simulink model "neckVel"  (Simulink 8.0)
settings: Solver=FixedStepDiscrete  StartTime=0.0  StopTime=inf  FixedStep=Ts  RelTol=1e-3
InitFcn:
  | initNeckVel;
undefined symbols (not defined in the file): DiscIntNeverNeededParam, DT, kCom, kImp, kw, qFin, Ts
libraries: WBCLibrary x36
settings Model: Creator=daniele  LastModifiedBy=icub
settings DebuggingCC: FcnCallInpInsideContextMsg=EnableAllAsWarning
settings CodeAppCC: CustomSymbolStrType=$N$R$M_T
settings GRTTargetCC: CodeReplacementLibrary=C89/C90 (ANSI)  CombineOutputUpdateFcns=off  GRTInterface=on

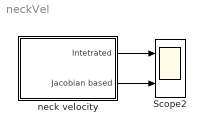
== system neckVel ==
  Scope2 : Scope  NumInputPorts=2
      settings: ShowLegends=on  YMin=-15~-5  YMax=70~5  SaveName=ScopeData2
  neck velocity : Subsystem  mask{robotName='icubGazeboSim', localName='simulink', Ts=Ts}
      mask prompts: robotName "Robot name"; localName "Local name"
  wires:
  neck velocity/1(Intetrated) -> Scope2/1
  neck velocity/2(Jacobian based) -> Scope2/2

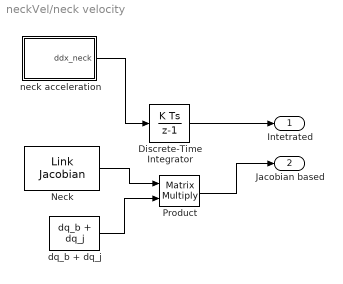
== system neckVel/neck velocity ==
  Discrete-Time Integrator : DiscreteIntegrator  InitialCondition=[0 0 0 0 0 0]  SampleTime=Ts  ICPrevOutput=DiscIntNeverNeededParam  ICPrevScaledInput=DiscIntNeverNeededParam
  Neck : WBCLibrary/wholeBodyModel/Jacobians/Link Jacobian  robotname=robotName  localname=localName  link=chest
  Product : Product  Multiplication=Matrix(*)  SampleTime=Ts  RndMeth=Zero
  dq_b + dq_j : WBCLibrary/wholeBodyStates/dq_b + dq_j  robotName=robotName  localName=localName  Ts=Ts
  neck acceleration : Subsystem  mask{robotName=robotName, localName=localName, Ts=0.010}
      mask prompts: robotName "Robot name"; localName "Local name"
  Intetrated : Outport
  Jacobian based : Outport  Port=2
  wires:
  dq_b + dq_j/1 -> Product/2
  Neck/1 -> Product/1
  Product/1 -> Jacobian based/1
  neck acceleration/1(ddx_neck) -> Discrete-Time Integrator/1
  Discrete-Time Integrator/1 -> Intetrated/1

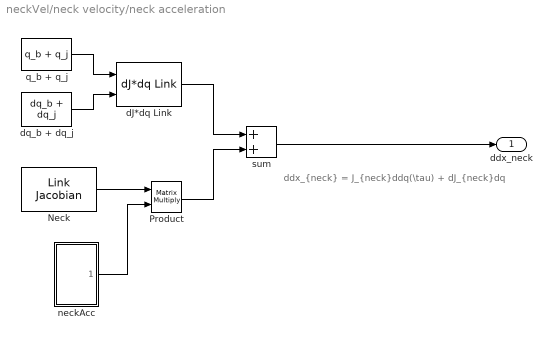
== system neckVel/neck velocity/neck acceleration ==
  note: ddx_{neck} = J_{neck}ddq(\tau) + dJ_{neck}dq
  Neck : WBCLibrary/wholeBodyModel/Jacobians/Link Jacobian  robotname=robotName  localname=localName  link=chest
  Product : Product  Multiplication=Matrix(*)  RndMeth=Zero
  dJ*dq Link : WBCLibrary/wholeBodyModel/Dynamics/dJ*dq Link  val=19  robotName=robotName  localName=localName  link=chest
  dq_b + dq_j : WBCLibrary/wholeBodyStates/dq_b + dq_j  robotName=robotName  localName=localName  Ts=Ts
  neckAcc : Subsystem  mask{robotName=robotName, Ts=Ts, localName=localName}
      mask prompts: robotName "robot name"; localName "module name"
  q_b + q_j : WBCLibrary/wholeBodyStates/q_b + q_j  robotName=robotName  localName=localName  Ts=Ts
  sum : Sum  SampleTime=Ts
  ddx_neck : Outport
  wires:
  dJ*dq Link/1 -> sum/1
  sum/1 -> ddx_neck/1
  q_b + q_j/1 -> dJ*dq Link/1
  neckAcc/1(ddq(tau)) -> Product/2
  Product/1 -> sum/2
  Neck/1 -> Product/1
  dq_b + dq_j/1 -> dJ*dq Link/2

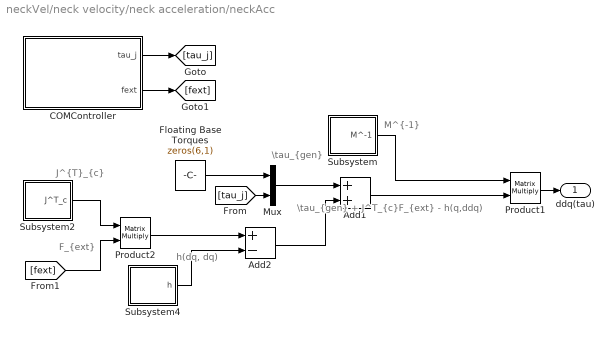
== system neckVel/neck velocity/neck acceleration/neckAcc ==
  note: \tau_{gen} + J^T_{c}F_{ext} - h(q,ddq)
  note: h(dq, dq)
  note: J^{T}_{c}
  note: M^{-1}
  note: F_{ext}
  note: \tau_{gen}
  Add1 : Sum  SampleTime=Ts
  Add2 : Sum  Inputs=+-  SampleTime=Ts
  COMController : Subsystem
  Floating Base Torques : Constant  Value=zeros(6,1)  SampleTime=Ts
  Mux : Mux  Inputs=2
  Product1 : Product  Multiplication=Matrix(*)  SampleTime=Ts
  Product2 : Product  Multiplication=Matrix(*)  SampleTime=Ts
  Subsystem : Subsystem
  Subsystem2 : Subsystem
  Subsystem4 : Subsystem
  ddq(tau) : Outport
  wires:
  Subsystem2/1(J^T_c) -> Product2/1
  [fext] -> Product2/2
  Product2/1 -> Add2/1
  Product1/1 -> ddq(tau)/1
  Add2/1 -> Add1/2
  Subsystem/1(M^-1) -> Product1/1
  Subsystem4/1(h) -> Add2/2
  Add1/1 -> Product1/2
  COMController/1(tau_j) -> [tau_j]
  COMController/2(fext) -> [fext]
  Floating Base Torques/1 -> Mux/1
  [tau_j] -> Mux/2
  Mux/1 -> Add1/1

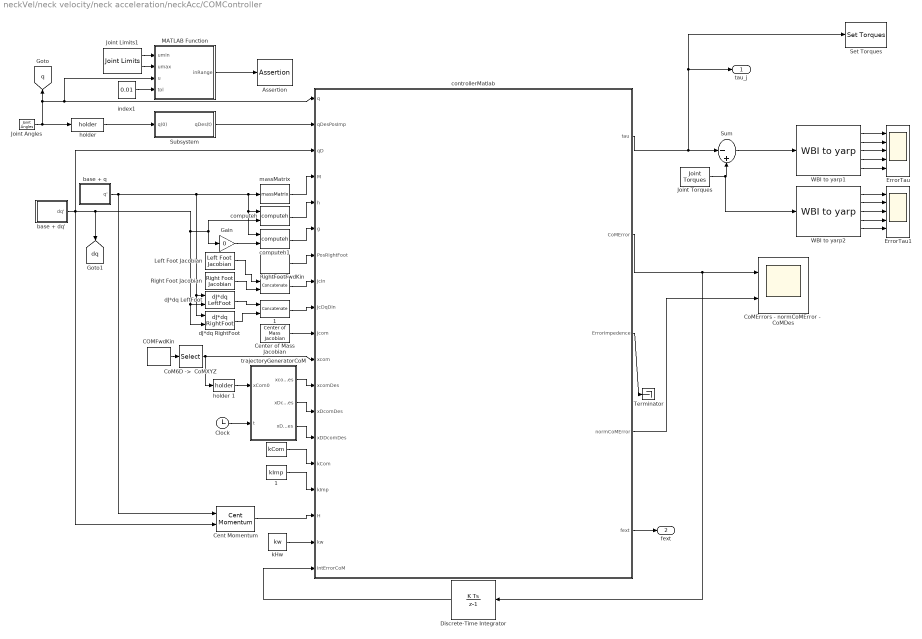
== system neckVel/neck velocity/neck acceleration/neckAcc/COMController ==
  "    " : Constant  Value=kCom
  "    1" : Constant  Value=kImp
  " " : Concatenate  Mode=Multidimensional array
  " 1" : Concatenate  Mode=Multidimensional array
  Assertion : Assertion  Enabled=on
  "COMFwdKin " : WBCLibrary/wholeBodyModel/Forward Kinematics/COMFwdKin   robotName=robotName  localName=localName
  Cent Momentum : WBCLibrary/wholeBodyModel/Dynamics/Cent Momentum  robotName=robotName  localName=localName
  Center of Mass Jacobian : WBCLibrary/wholeBodyModel/Jacobians/Center of Mass Jacobian  robotName=robotName  localName=localName
  Clock : Clock
  "CoM6D ->  CoMXYZ" : Selector  InputPortWidth=7  IndexOptions=Index vector (dialog)  Indices=[1 2 3]  OutputSizes=1
  "CoMErrors - normCoMError -   CoMDes " : Scope  NumInputPorts=2
      settings: TimeRange=0.5  YMin=-0.025~0  YMax=0.005~0.04  SaveName=ScopeData6
  Discrete-Time Integrator : DiscreteIntegrator  InitialCondition=[0 0 0]  SampleTime=Ts  ICPrevOutput=DiscIntNeverNeededParam  ICPrevScaledInput=DiscIntNeverNeededParam
  ErrorTau : Scope  NumInputPorts=5
      settings: ShowLegends=on  YMin=-12~-5~-5~-5~-5  YMax=12~5~5~5~5
  ErrorTau1 : Scope  NumInputPorts=5
      settings: YMin=-12~-5~-5~-5~-5  YMax=12~5~5~5~5
  Gain : Gain  Gain=0
  Joint Angles : WBCLibrary/wholeBodyStates/Joint Angles  robotName=robotName  localName=localName
  Joint Limits1 : WBCLibrary/wholeBodyModel/Joint Limits  robotName=robotName  localName=localName
  Joint Torques : WBCLibrary/wholeBodyStates/Joint Torques  robotName=robotName  localName=localName
  Left Foot Jacobian : WBCLibrary/wholeBodyModel/Jacobians/Left Foot Jacobian  robotName=robotName  localName=localName
  MATLAB Function : MATLAB Function  TreatAsAtomicUnit=on
  Right Foot Jacobian : WBCLibrary/wholeBodyModel/Jacobians/Right Foot Jacobian  robotName=robotName  localName=localName
  RightFootFwdKin : WBCLibrary/wholeBodyModel/Forward Kinematics/RightFootFwdKin  robotName=robotName  localName=localName
  Set Torques : WBCLibrary/wholeBodyActuators/Set Torques  val=6  robotName=robotName  localName=localName
  Subsystem : Subsystem
  Sum : Sum  Inputs=|-+
  Terminator : Terminator
  WBI to yarp1 : WBCLibrary/Utilities/WBI to yarp
  WBI to yarp2 : WBCLibrary/Utilities/WBI to yarp
  base + dq' : Subsystem
  base + q : Subsystem
  computeh : WBCLibrary/wholeBodyModel/Dynamics/computeh  val=7  robotname=robotName  localname=localName
  computeh1 : WBCLibrary/wholeBodyModel/Dynamics/computeh  val=7  robotname=robotName  localname=localName
  controllerMatlab : MATLAB Function  TreatAsAtomicUnit=on
  dJ*dq LeftFoot : WBCLibrary/wholeBodyModel/Dynamics/dJ*dq LeftFoot  val=9  robotName=robotName  localName=localName
  dJ*dq RightFoot : WBCLibrary/wholeBodyModel/Dynamics/dJ*dq RightFoot  val=9  robotName=robotName  localName=localName
  "holder " : WBCLibrary/Utilities/holder 
  holder 1 : WBCLibrary/Utilities/holder 
  index1 : Constant  Value=0.01  VectorParams1D=off
  kHw : Constant  Value=kw
  massMatrix : WBCLibrary/wholeBodyModel/Dynamics/massMatrix  val=8  robotname=robotName  localname=localName
  trajectoryGeneratorCoM : MATLAB Function  TreatAsAtomicUnit=on
  tau_j : Outport
  fext : Outport  Port=2
  tag scope: dq=global, q=global
  wires:
  computeh/1 -> controllerMatlab/5(h)
  " "/1 -> controllerMatlab/8(JcIn)
  dJ*dq RightFoot/1 -> " 1"/2
  "    1"/1 -> controllerMatlab/16(kImp)
  kHw/1 -> controllerMatlab/18(kw)
  Joint Torques/1 -> WBI to yarp2/1, Sum/2
  WBI to yarp2/2 -> ErrorTau1/2
  MATLAB Function/1(inRange) -> Assertion/1
  "    "/1 -> controllerMatlab/15(kCom)
  WBI to yarp1/5 -> ErrorTau/5
  "CoM6D ->  CoMXYZ"/1 -> holder 1/1, controllerMatlab/11(xcom)
  base + q/1(q') -> dJ*dq RightFoot/1, dJ*dq LeftFoot/1, computeh1/1, computeh/1, massMatrix/1, Cent Momentum/1
  dJ*dq LeftFoot/1 -> " 1"/1
  base + dq'/1(dq') -> [dq], dJ*dq RightFoot/2, dJ*dq LeftFoot/2, computeh/2, Gain/1, Cent Momentum/2, controllerMatlab/3(qD)
  index1/1 -> MATLAB Function/4(tol)
  Joint Limits1/1 -> MATLAB Function/1(umin)
  "holder "/1 -> Subsystem/1(q(0))
  Gain/1 -> computeh1/2
  trajectoryGeneratorCoM/3(xDDcomDes) -> controllerMatlab/14(xDDcomDes)
  Subsystem/1(qDes(t)) -> controllerMatlab/2(qDesPosImp)
  WBI to yarp2/1 -> ErrorTau1/1
  computeh1/1 -> controllerMatlab/6(g)
  Joint Limits1/2 -> MATLAB Function/2(umax)
  WBI to yarp1/2 -> ErrorTau/2
  holder 1/1 -> trajectoryGeneratorCoM/1(xCom0)
  Clock/1 -> trajectoryGeneratorCoM/2(t)
  "COMFwdKin "/1 -> "CoM6D ->  CoMXYZ"/1
  Sum/1 -> WBI to yarp1/1
  trajectoryGeneratorCoM/1(xcomDes) -> controllerMatlab/12(xcomDes)
  Left Foot Jacobian/1 -> " "/1
  WBI to yarp2/4 -> ErrorTau1/4
  WBI to yarp1/3 -> ErrorTau/3
  massMatrix/1 -> controllerMatlab/4(M)
  WBI to yarp1/4 -> ErrorTau/4
  RightFootFwdKin/1 -> controllerMatlab/7(PosRightFoot)
  controllerMatlab/1(tau) -> tau_j/1, Set Torques/1, Sum/1
  trajectoryGeneratorCoM/2(xDcomDes) -> controllerMatlab/13(xDcomDes)
  Discrete-Time Integrator/1 -> controllerMatlab/19(IntErrorCoM)
  WBI to yarp1/1 -> ErrorTau/1
  Joint Angles/1 -> MATLAB Function/3(u), controllerMatlab/1(q), [q], "holder "/1
  WBI to yarp2/3 -> ErrorTau1/3
  controllerMatlab/4(normCoMError) -> "CoMErrors - normCoMError -   CoMDes "/2
  " 1"/1 -> controllerMatlab/9(JcDqDIn)
  Cent Momentum/1 -> controllerMatlab/17(H)
  controllerMatlab/2(CoMError) -> Discrete-Time Integrator/1, "CoMErrors - normCoMError -   CoMDes "/1
  controllerMatlab/3(ErrorImpedence) -> Terminator/1
  Center of Mass Jacobian/1 -> controllerMatlab/10(Jcom)
  Right Foot Jacobian/1 -> " "/2
  WBI to yarp2/5 -> ErrorTau1/5
  controllerMatlab/5(fext) -> fext/1

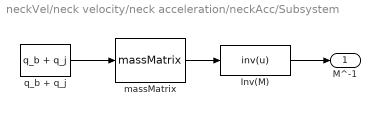
== system neckVel/neck velocity/neck acceleration/neckAcc/Subsystem ==
  Inv(M) : MATLABFcn  MATLABFcn=inv(u)  Output1D=off  SampleTime=Ts
  massMatrix : WBCLibrary/wholeBodyModel/Dynamics/massMatrix  val=8  robotname=robotName  localname=localName
  q_b + q_j : WBCLibrary/wholeBodyStates/q_b + q_j  robotName=robotName  localName=localName  Ts=Ts
  M^-1 : Outport
  wires:
  q_b + q_j/1 -> massMatrix/1
  Inv(M)/1 -> M^-1/1
  massMatrix/1 -> Inv(M)/1

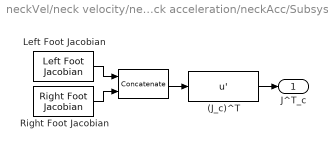
== system neckVel/neck velocity/neck acceleration/neckAcc/Subsystem2 ==
  " " : Concatenate  Mode=Multidimensional array
  (J_c)^T : MATLABFcn  MATLABFcn=u'  Output1D=off  SampleTime=Ts
  Left Foot Jacobian : WBCLibrary/wholeBodyModel/Jacobians/Left Foot Jacobian  robotName=robotName  localName=localName
  Right Foot Jacobian : WBCLibrary/wholeBodyModel/Jacobians/Right Foot Jacobian  robotName=robotName  localName=localName
  J^T_c : Outport
  wires:
  (J_c)^T/1 -> J^T_c/1
  " "/1 -> (J_c)^T/1
  Right Foot Jacobian/1 -> " "/2
  Left Foot Jacobian/1 -> " "/1

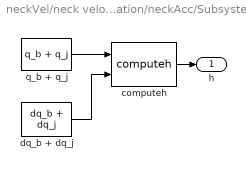
== system neckVel/neck velocity/neck acceleration/neckAcc/Subsystem4 ==
  computeh : WBCLibrary/wholeBodyModel/Dynamics/computeh  val=7  robotname=robotName  localname=localName
  dq_b + dq_j : WBCLibrary/wholeBodyStates/dq_b + dq_j  robotName=robotName  localName=localName  Ts=Ts
  q_b + q_j : WBCLibrary/wholeBodyStates/q_b + q_j  robotName=robotName  localName=localName  Ts=Ts
  h : Outport
  wires:
  computeh/1 -> h/1
  q_b + q_j/1 -> computeh/1
  dq_b + dq_j/1 -> computeh/2

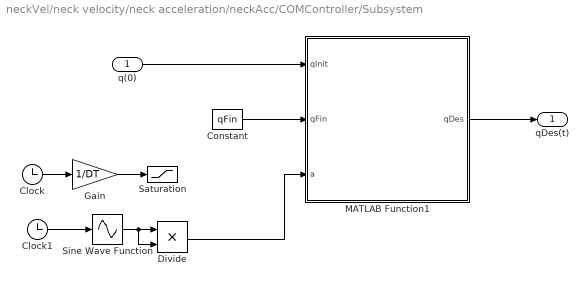
== system neckVel/neck velocity/neck acceleration/neckAcc/COMController/Subsystem ==
  q(0) : Inport
  Clock : Clock
  Clock1 : Clock
  Constant : Constant  Value=qFin
  Divide : Product  Inputs=**
  Gain : Gain  Gain=1/DT
  MATLAB Function1 : MATLAB Function  TreatAsAtomicUnit=on
  Saturation : Saturate  UpperLimit=1  LowerLimit=0  SampleTime=Ts
  Sine Wave Function : Sin  TimeSource=Use external signal  Frequency=pi/DT  SampleTime=0
  qDes(t) : Outport
  wires:
  q(0)/1 -> MATLAB Function1/1(qInit)
  MATLAB Function1/1(qDes) -> qDes(t)/1
  Constant/1 -> MATLAB Function1/2(qFin)
  Clock/1 -> Gain/1
  Gain/1 -> Saturation/1
  Clock1/1 -> Sine Wave Function/1
  Sine Wave Function/1 -> Divide/2, Divide/1
  Divide/1 -> MATLAB Function1/3(a)

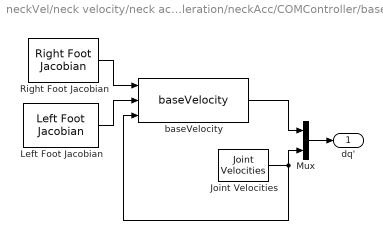
== system neckVel/neck velocity/neck acceleration/neckAcc/COMController/base + dq' ==
  Joint Velocities : WBCLibrary/wholeBodyStates/Joint Velocities  robotName=robotName  localName=localName
  Left Foot Jacobian : WBCLibrary/wholeBodyModel/Jacobians/Left Foot Jacobian  robotName=robotName  localName=localName
  Mux : Mux  Inputs=2
  Right Foot Jacobian : WBCLibrary/wholeBodyModel/Jacobians/Right Foot Jacobian  robotName=robotName  localName=localName
  baseVelocity : WBCLibrary/Utilities/baseVelocity
  dq' : Outport
  wires:
  Left Foot Jacobian/1 -> baseVelocity/2
  Right Foot Jacobian/1 -> baseVelocity/1
  baseVelocity/1 -> Mux/1
  Joint Velocities/1 -> baseVelocity/3, Mux/2
  Mux/1 -> dq'/1

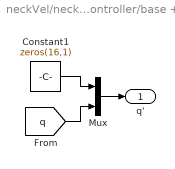
== system neckVel/neck velocity/neck acceleration/neckAcc/COMController/base + q ==
  Constant1 : Constant  Value=zeros(16,1)
  Mux : Mux  Inputs=2
  q' : Outport
  wires:
  Mux/1 -> q'/1
  [q] -> Mux/2
  Constant1/1 -> Mux/1

== matlab function neck velocity/neck acceleration/neckAcc/COMController/trajectoryGeneratorCoM ==
  data: xcomDes output double; xDcomDes output double; xDDcomDes output double; xCom0 input double; t input double
function [xcomDes, xDcomDes, xDDcomDes] = fcn(xCom0,t)
%#codegen

e3 = [0;1;0];
A = 0.01;%15;
f = 0.15;

xcomDes    = xCom0 + A*sin(2*pi*f*t)*e3;
xcomDes(3) =  xcomDes(3) + 0.01;
xDcomDes   =         A*2*pi*f*cos(2*pi*f*t)*e3;
xDDcomDes  =        -A*(2*pi*f)^2*sin(2*pi*f*t)*e3;

== matlab function neck velocity/neck acceleration/neckAcc/COMController/controllerMatlab ==
  data: q input double; qDesPosImp input double; qD input double; M input double; h input double; g input double; PosRightFoot input double; JcIn input double; JcDqDIn input double; tau output double; Jcom input double; xcom input double; xcomDes input double; xDcomDes input double; xDDcomDes input double; kCom input double; kImp input double; H input double; kw input double; CoMError output double; IntErrorCoM input double; ErrorImpedence output double; normCoMError output double; fext output double
function [tau,CoMError,ErrorImpedence,normCoMError,fext] = fcn(q,qDesPosImp,qD, M, h, g, PosRightFoot, JcIn, JcDqDIn, Jcom, xcom, xcomDes, xDcomDes, xDDcomDes, kCom, kImp ,H, kw,IntErrorCoM)
%#codegen

PINV_TOL = 1e-5;
gravAcc        = 9.81;

n = 25;
St    = [zeros(6,n);eye(n,n)];

m     = M(1,1);
grav = [zeros(2,1);-m*gravAcc;zeros(3,1)];

% Definition of reference accelerations for CoM and Joints that ensure
% stabilization of desired trajectories xDcomDes and qDes 

xDcom      = Jcom(1:3,:)*qD;
xDDcomStar = xDDcomDes - kCom(1)*(xcom - xcomDes) - kCom(2)*IntErrorCoM - kCom(3)*(xDcom - xDcomDes)  ;

Pr =  PosRightFoot(1:3) - xcom; % Application point of the contact force on the right foot w.r.t. CoM

A  = [ eye(3),   zeros(3),eye(3), zeros(3);
      -Sf(xcom),  eye(3), Sf(Pr), eye(3) ];
hwDotDes = H(4:end);
hDotDes  = [ m*xDDcomStar ;
             -kw*hwDotDes  ]; 
Jc = JcIn;         
JcDqD = JcDqDIn;

% Jc    = [JcIn(1:3,:);JcIn(7:9,:)];       
% JcDqD = [JcDqDIn(1:3,:);JcDqDIn(7:9,:)];

% A  = [ eye(3),eye(3)];
% hDotDes  =  m*xDDcomStar; 
% fextMeas = [fextMeasIn(1:3);fextMeasIn(7:9)];

pinvA = pinv(A, PINV_TOL);
fd    = pinvA*(hDotDes-grav) ;% + (eye(length(fext)) - pinvA*A)*fext;

Minv = inv(M);
JcMinv        = Jc*Minv;
PInv_JcMinvSt = pinv(JcMinv*St, PINV_TOL);
N0            = eye(n) - PInv_JcMinvSt*JcMinv*St;

fext = fd;

tau1 = PInv_JcMinvSt*(JcMinv*h - JcDqD - JcMinv*Jc'*fd);
LinearizedDynamics = g(7:end)-Jc(:,7:end)'*fext - kImp.*(q-qDesPosImp);% - tau1 -diag(kDam)*N0'*qD(7:end) ;  %-kDam.*qD(7:end) 

tau0 = LinearizedDynamics;

tau = tau1 + N0*tau0;

% f = (JcMinv*Jc')^-1*(JcMinv*(h-[zeros(6,1);tau])-JcDqD);

CoMError    = xcom - xcomDes;
normCoMError  = norm(CoMError);
ErrorImpedence   = tau + LinearizedDynamics;

== matlab function neck velocity/neck acceleration/neckAcc/COMController/Subsystem/MATLAB Function1 ==
  data: qInit input double; qFin input double; qDes output double; a input double
function qDes = checkRange(qInit,qFin,a)
%#codegen
 
qFin(qFin == -5) = qInit(qFin == -5);

qDes = qInit + a*(qFin-qInit);

== matlab function neck velocity/neck acceleration/neckAcc/COMController/MATLAB Function ==
  data: umin input double; umax input double; u input double; inRange output double; tol input double
function inRange = checkRange(umin, umax, u, tol)
%#codegen

res = u < umin + tol | u > umax - tol;
res = sum(res);
if res==0
    inRange = 1;
else
    inRange = 0;
    u < umin + tol | u > umax - tol
end
